simulink model "ex2_HW4_Boeru"  (R2017b)
settings: Solver=FixedStepAuto  StartTime=0.0  StopTime=0.0006  FixedStep=0.0000002  RelTol=1e-3
settings Model: Creator=Iva  LastModifiedBy=Briana

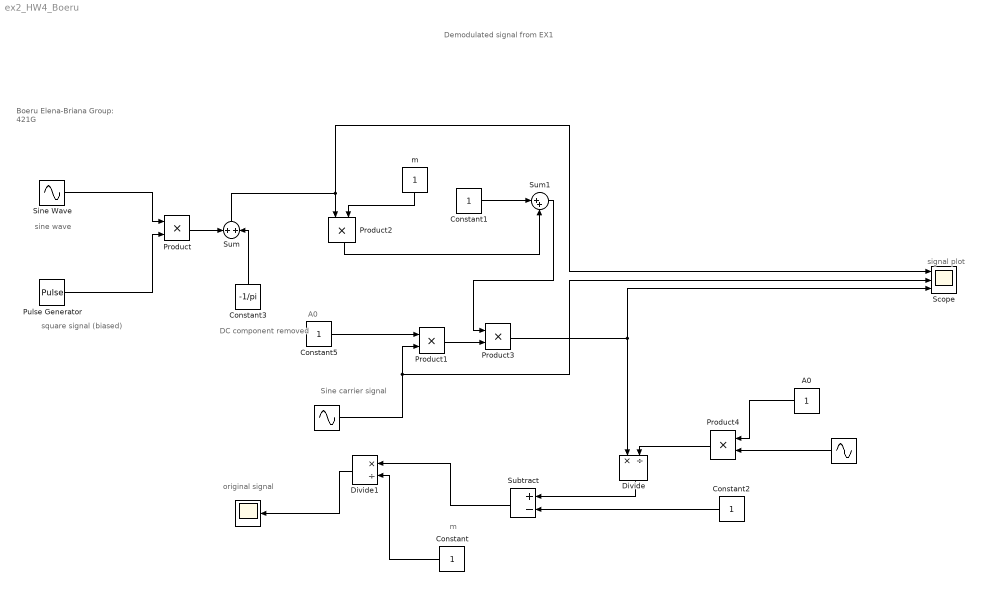
== system ex2_HW4_Boeru ==
  note: Demodulated signal from EX1
  note: Boeru Elena-Briana
      | Group: 421G
  note: square signal (biased)
  note: sine wave
  note: DC component
      | removed
  note: Sine carrier signal
  note: A0
  note: signal plot
  note: original signal
  note: m
  " " : Scope
  " " : Sin  Frequency=2*pi*500000  SampleTime=0
  " " : Sin  Frequency=2*pi*500000  SampleTime=0
  A0 : Constant
  Constant{,1..2,5} (4 alike) : Constant
  Constant3 : Constant  Value=-1/pi
  Divide : Product  Inputs=*/
  Divide1 : Product  Inputs=*/
  Product{,1..4} (5 alike) : Product
  Pulse Generator : DiscretePulseGenerator  PulseType=Time based  Period=0.0002  PulseWidth=50
  Scope : Scope  NumInputPorts=3
  Sine Wave : Sin  Frequency=2*pi*5000  SampleTime=0
  Subtract : Sum  Inputs=+-
  Sum : Sum  Inputs=2
  Sum1 : Sum  Inputs=|++
  m : Constant
  wires:
  Sine Wave/1 -> Product/1
  Pulse Generator/1 -> Product/2
  Constant3/1 -> Sum/2
  Product/1 -> Sum/1
  Sum/1 -> Product2/1, Scope/1
  m/1 -> Product2/2
  Product2/1 -> Sum1/2
  Constant1/1 -> Sum1/1
  Sum1/1 -> Product3/1
  Product1/1 -> Product3/2
  Product3/1 -> Scope/3, Divide/1
  Constant5/1 -> Product1/1
  " "/1 -> Product1/2, Scope/2
  Divide/1 -> Subtract/1
  Subtract/1 -> Divide1/1
  Divide1/1 -> " "/1
  Product4/1 -> Divide/2
  A0/1 -> Product4/1
  " "/1 -> Product4/2
  Constant2/1 -> Subtract/2
  Constant/1 -> Divide1/2
